simulink model "Dougherty1968_Linear_Paper-Approximation"  (R2022b)
settings: Solver=ode45  StartTime=0.0  StopTime=5000.0  MaxStep=200.0  RelTol=1e-3
model workspace (MAT data in the model file):
  Ix = 1000
  Ixy = 0
  Ixz = 0
  Iy = 250
  Iyz = 0
  Iz = 1000
  K_i = 1150
  K_p = 25
  T_c = 1
  T_c_x = 0
  T_c_z = 0
  T_d_x = 0
  T_d_z = 0
  h = 150
  k_phi = 46
  offset = 0.0175
  omega_0 = 7.3e-05
  phi_0 = 0.0175
  phi_d = 10
  psi_0 = 0
  tau = 25
libraries: simulink_extras x2
settings Model: Creator=Kirtan  LastModifiedBy=Kirtan

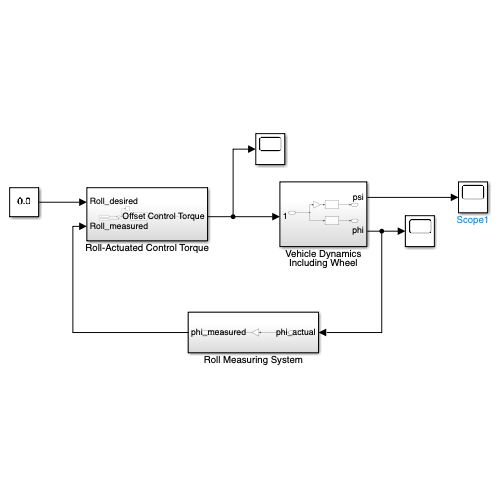
[thumbnail: Simulink's stored preview of the top-level diagram]
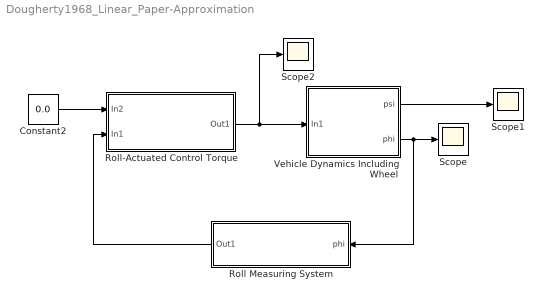
== system Dougherty1968_Linear_Paper-Approximation ==
  Constant2 : Constant  Value=0.0
  Roll Measuring System : Subsystem
  Roll-Actuated Control Torque : Subsystem
  Scope : Scope
  Scope1 : Scope
  Scope2 : Scope
  Vehicle Dynamics Including Wheel : Subsystem
  wires:
  Roll Measuring System/1(Out1) -> Roll-Actuated Control Torque/2(In1)
  Constant2/1 -> Roll-Actuated Control Torque/1(In2)
  Vehicle Dynamics Including Wheel/2(phi) -> Roll Measuring System/1(phi), Scope/1
  Roll-Actuated Control Torque/1(Out1) -> Scope2/1, Vehicle Dynamics Including Wheel/1(In1)
  Vehicle Dynamics Including Wheel/1(psi) -> Scope1/1

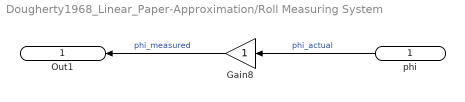
== system Dougherty1968_Linear_Paper-Approximation/Roll Measuring System ==
  phi : Inport
  Gain8 : Gain
  Out1 : Outport
  wires:
  Gain8/1 -> Out1/1  "phi_measured"
  phi/1 -> Gain8/1  "phi_actual"

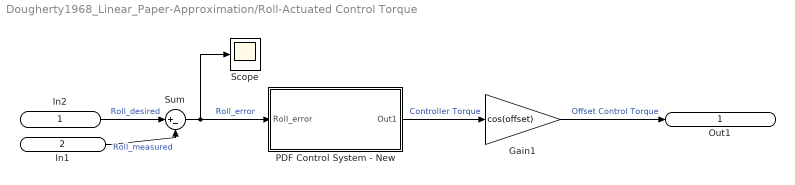
== system Dougherty1968_Linear_Paper-Approximation/Roll-Actuated Control Torque ==
  In2 : Inport
  In1 : Inport  Port=2
  Gain1 : Gain  Gain=cos(offset)
  PDF Control System - New : Subsystem
  Scope : Scope
  Sum : Sum  Inputs=|+-
  Out1 : Outport
  wires:
  In1/1 -> Sum/2  "Roll_measured"
  In2/1 -> Sum/1  "Roll_desired"
  Sum/1 -> PDF Control System - New/1(Roll_error), Scope/1  "Roll_error"
  PDF Control System - New/1(Out1) -> Gain1/1  "Controller Torque"
  Gain1/1 -> Out1/1  "Offset Control Torque"

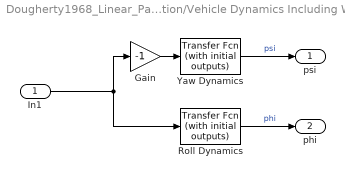
== system Dougherty1968_Linear_Paper-Approximation/Vehicle Dynamics Including Wheel ==
  In1 : Inport
  Gain : Gain  Gain=-1
  Roll Dynamics : simulink_extras/Additional Linear/Transfer Fcn (with initial outputs)  N=[Iz h*tan(offset) omega_0*h]  D=[Ix*Iz 0 (h*h + Ix*Iz*omega_0*omega_0) 0 (h*h*omega_0*omega_0)]  Y0=.0175  U0=0
  Yaw Dynamics : simulink_extras/Additional Linear/Transfer Fcn (with initial outputs)  N=[Ix*tan(offset) -1*h omega_0*h*tan(offset)]  D=[Ix*Iz 0 (h*h + Ix*Iz*omega_0*omega_0) 0 (h*h*omega_0*omega_0)]  Y0=0.0175  U0=0
  psi : Outport
  phi : Outport  Port=2
  wires:
  Yaw Dynamics/1 -> psi/1  "psi"
  Roll Dynamics/1 -> phi/1  "phi"
  In1/1 -> Roll Dynamics/1, Gain/1
  Gain/1 -> Yaw Dynamics/1

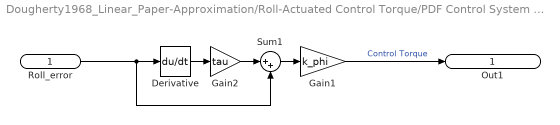
== system Dougherty1968_Linear_Paper-Approximation/Roll-Actuated Control Torque/PDF Control System - New ==
  Roll_error : Inport
  Derivative : Derivative
  Gain1 : Gain  Gain=k_phi
  Gain2 : Gain  Gain=tau
  Sum1 : Sum  Inputs=|++
  Out1 : Outport
  wires:
  Gain2/1 -> Sum1/1
  Roll_error/1 -> Sum1/2, Derivative/1
  Derivative/1 -> Gain2/1
  Gain1/1 -> Out1/1  "Control Torque"
  Sum1/1 -> Gain1/1
